simulink model "TorqueVectoring_6_1"  (R2023a)
settings: Solver=FixedStepAuto  StartTime=0.0  StopTime=8  FixedStep=.001  RelTol=1e-3
model workspace (MAT data in the model file):
  slipTarget : Simulink.Parameter (value not decoded)
values from neighbouring files (symbols this model uses):
  Kd_slip = 0    [Main_TorqueVectoring_5_1.m]
  Kd_yaw = 0    [Main_TorqueVectoring_5_1.m]
  Ki_slip = 50    [Main_TorqueVectoring_5_1.m]
  Ki_yaw = 10    [Main_TorqueVectoring_5_1.m]
  Kp_slip = 250    [Main_TorqueVectoring_5_1.m]
  Kp_yaw = 100    [Main_TorqueVectoring_5_1.m]
  slip_windupLower = -inf    [Main_TorqueVectoring_5_1.m]
  slip_windupUpper = inf    [Main_TorqueVectoring_5_1.m]
  slipTarget = .2    (= 0.2)    [Main_TorqueVectoring_5_1.m]
  steering = table2array(yawrateSteering)    [Main_TorqueVectoring_5_1.m]
  yaw_prev_error = 0    [Main_TorqueVectoring_5_1.m]
  yawRate = table2array(yawrateTable)    [Main_TorqueVectoring_5_1.m]
  yawrateVelocity = [0, 5, 10, 15, 20, 25, 30, 35]    [Main_TorqueVectoring_5_1.m]
undefined symbols (not defined in the file or in its folder): sigbuilder_block, VehicleVelocity
libraries: slpidlib x6
(part 4 of 4)

== matlab function TorqueVectoring_6_1/Vehicle Dynamics Model/14 DOF MODEL/Subsys Tire/Subsys tfl3/Fy Tire ==
  data: SA input; FY output; FZ input
function FY  = FYgen_H16x75LC07(SA, FZ)
%{
Coefficient values for tire are obtained through tire parser
c(1) = a0
c(2) = a1
.... etc
%}

c = [1.3662,0.0013,2.7913,7322.2407,300.0032,0.3242];
a0 = c(1);
a1 = c(2);
a2 = c(3);
a3 = c(4);
a4 = c(5);
a7 = c(6); 

C = a0;
H = 0;
E = a7;
V = 0;

D = FZ.*(a1.*FZ+a2);
BCD = a3.*sin(atan(FZ./a4).*2);
B = BCD./(C.*D);
Bx1 = B.*(SA+H);

FY = D.*sin(C.*atan(Bx1-E.*(Bx1-atan(Bx1))))+V;
end

== matlab function TorqueVectoring_6_1/Traction Control/FL/MATLAB Function ==
  data: enable output; actualSlip input; setpoint output; SlipTarget input
function [enable,setpoint] = slipCtrlTrigger(actualSlip,SlipTarget)


if actualSlip >= 0 %Positive slip (Acceleration control)
    if actualSlip > SlipTarget 
        setpoint = SlipTarget;
        enable = 1; % Slip Control is active
    else 
        setpoint = 0; %Can this be commented out or does it need a value
                        %when disabled
        enable = 0;
    end

elseif actualSlip < 0 %Negative slip (Braking control)
    if actualSlip < SlipTarget*-1        
        setpoint = SlipTarget*-1;
        enable = 1; 
    else
        setpoint= 0;
        enable = 0;
    end
else
    setpoint = 0;
    enable = 0;
end

== matlab function TorqueVectoring_6_1/Traction Control/FR/MATLAB Function ==
  data: enable output; actualSlip input; setpoint output; SlipTarget input
function [enable,setpoint] = slipCtrlTrigger(actualSlip,SlipTarget)


if actualSlip >= 0 %Positive slip (Acceleration control)
    if actualSlip > SlipTarget 
        setpoint = SlipTarget;
        enable = 1; % Slip Control is active
    else 
        setpoint = 0; %Can this be commented out or does it need a value
                        %when disabled
        enable = 0;
    end

elseif actualSlip < 0 %Negative slip (Braking control)
    if actualSlip < SlipTarget*-1        
        setpoint = SlipTarget*-1;
        enable = 1; 
    else
        setpoint= 0;
        enable = 0;
    end
else
    setpoint = 0;
    enable = 0;
end
